simulink model "Simulacion"  (R2022b)
settings: Solver=VariableStepAuto  StartTime=0.0  StopTime=30  RelTol=1e-3
undefined symbols (not defined in the file): a, b, beta, J, Km, La, Ra
libraries: spsRMSLib x1
settings Model: Creator=danie  LastModifiedBy=danie

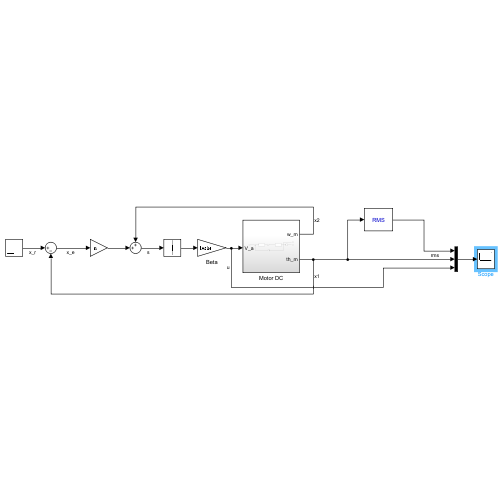
[thumbnail: Simulink's stored preview of the top-level diagram]
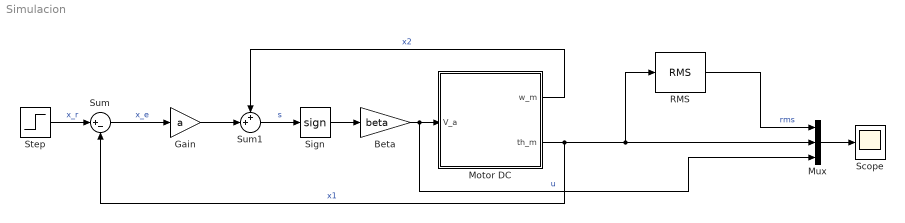
== system Simulacion ==
  Beta : Gain  Gain=beta
  Gain : Gain  Gain=a
  Motor DC : Subsystem
  Mux : Mux  Inputs=3
  RMS : spsRMSLib/RMS  TrueRMS=on  Freq=1/0.73  RMSInit=120  Ts=0
  Scope : Scope
  Sign : Signum
  Step : Step  SampleTime=0
  Sum : Sum  Inputs=|+-
  Sum1 : Sum  Inputs=++|
  wires:
  Motor DC/1(w_m) -> Sum1/1  "x2"
  Motor DC/2(th_m) -> Sum/2, RMS/1, Mux/2  "x1"
  Step/1 -> Sum/1  "x_r"
  Sum/1 -> Gain/1  "x_e"
  Gain/1 -> Sum1/2
  Sum1/1 -> Sign/1  "s"
  Beta/1 -> Mux/3, Motor DC/1(V_a)  "u"
  Sign/1 -> Beta/1
  RMS/1 -> Mux/1  "rms"
  Mux/1 -> Scope/1

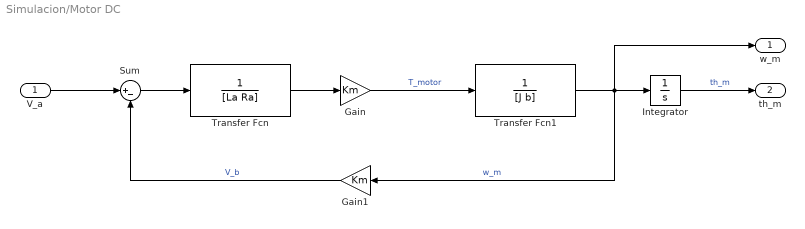
== system Simulacion/Motor DC ==
  V_a : Inport
  Gain : Gain  Gain=Km
  Gain1 : Gain  Gain=Km
  Integrator : Integrator
  Sum : Sum  Inputs=|+-
  Transfer Fcn : TransferFcn  Denominator=[La Ra]
  Transfer Fcn1 : TransferFcn  Denominator=[J b]
  w_m : Outport
  th_m : Outport  Port=2
  wires:
  Gain/1 -> Transfer Fcn1/1  "T_motor"
  Gain1/1 -> Sum/2  "V_b"
  Transfer Fcn1/1 -> w_m/1, Gain1/1, Integrator/1  "w_m"
  Transfer Fcn/1 -> Gain/1
  Integrator/1 -> th_m/1  "th_m"
  V_a/1 -> Sum/1
  Sum/1 -> Transfer Fcn/1
